simulink model "model_Zbiornik_wsk"  (R2015a)
settings: Solver=ode4  StartTime=0.0  StopTime=100.0  FixedStep=0.01  RelTol=1e-3
values from neighbouring files (symbols this model uses):
  h0 = 20    [NastawyLQR.m]    (also in SzukanieNastaw.m; wskaznikJakosci.m)
  pompaP1 = p1    [SzukanieNastaw.m]
  pompaPWM = ur(1)    [NastawyLQR.m]    (also in SzukanieNastaw.m; SzukanieStanuUstalonego.m = Nastawy(1); wskaznikJakosci.m = params(1))
  ref = 20    [wskaznikJakosci.m]
  zaworP1 = [-49.1428571429 99.1142857143 -23.37]    [parametryWielomianuPWMZaworu.mat]
  zaworPWM = ur(2)    [NastawyLQR.m]    (also in SzukanieNastaw.m; SzukanieStanuUstalonego.m = Nastawy(2); wskaznikJakosci.m = params(2))
undefined symbols (not defined in the file or in its folder): zaworC1, zaworC2
settings Model: Creator=konra  LastModifiedBy=konra

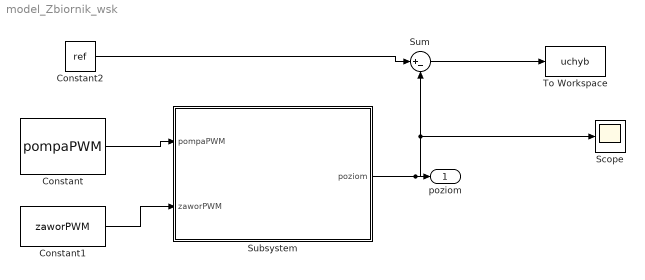
== system model_Zbiornik_wsk ==
  Constant : Constant  Value=pompaPWM
  Constant1 : Constant  Value=zaworPWM
  Constant2 : Constant  Value=ref
  Scope : Scope
      settings: TimeRange=49.99  YMin=19.999999925  YMax=19.999999965
  Subsystem : Subsystem
  Sum : Sum  Inputs=|+-
  To Workspace : ToWorkspace  VariableName=uchyb  SaveFormat=Structure With Time  SampleTime=-1
  poziom : Outport
  wires:
  Subsystem/1(poziom) -> Sum/2, Scope/1, poziom/1
  Constant/1 -> Subsystem/1(pompaPWM)
  Constant1/1 -> Subsystem/2(zaworPWM)
  Constant2/1 -> Sum/1
  Sum/1 -> To Workspace/1

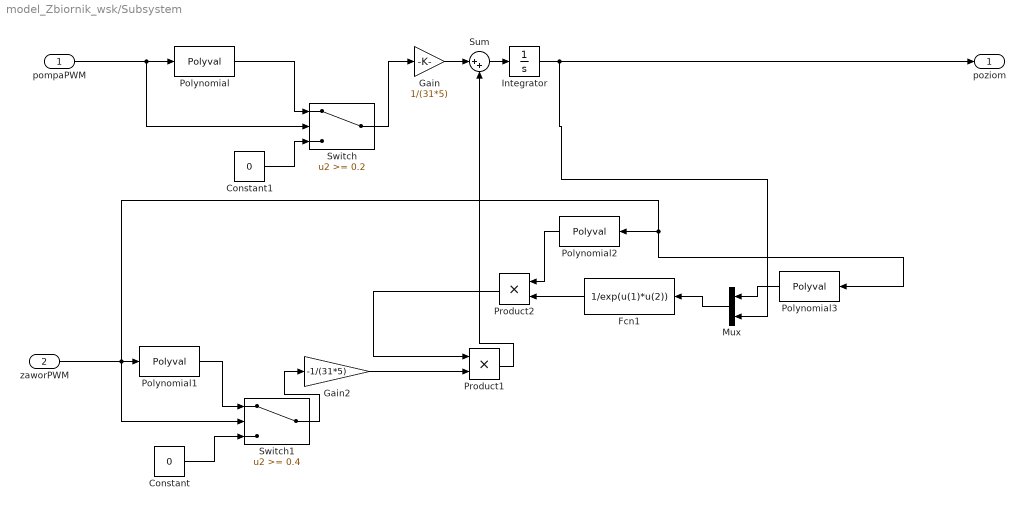
== system model_Zbiornik_wsk/Subsystem ==
  pompaPWM : Inport
  zaworPWM : Inport  Port=2
  Constant : Constant  Value=0
  Constant1 : Constant  Value=0
  Fcn1 : Fcn  Expr=1/exp(u(1)*u(2))
  Gain : Gain  Gain=1/(31*5)
  Gain2 : Gain  Gain=-1/(31*5)
  Integrator : Integrator  InitialCondition=h0
  Mux : Mux  Inputs=2
  Polynomial : Polyval  Coefs=pompaP1
  Polynomial1 : Polyval  Coefs=zaworP1
  Polynomial2 : Polyval  Coefs=zaworC2
  Polynomial3 : Polyval  Coefs=zaworC1
  Product1 : Product
  Product2 : Product
  Sum : Sum  Inputs=|++
  Switch : Switch  Threshold=0.2
  Switch1 : Switch  Threshold=0.4
  poziom : Outport
  wires:
  Switch1/1 -> Gain2/1
  Polynomial1/1 -> Switch1/1
  Constant/1 -> Switch1/3
  Polynomial/1 -> Switch/1
  Constant1/1 -> Switch/3
  Switch/1 -> Gain/1
  pompaPWM/1 -> Switch/2, Polynomial/1
  Gain2/1 -> Product1/2
  Product1/1 -> Sum/2
  Product2/1 -> Product1/1
  Integrator/1 -> poziom/1, Mux/2
  Fcn1/1 -> Product2/2
  zaworPWM/1 -> Switch1/2, Polynomial1/1, Polynomial3/1, Polynomial2/1
  Polynomial2/1 -> Product2/1
  Mux/1 -> Fcn1/1
  Polynomial3/1 -> Mux/1
  Gain/1 -> Sum/1
  Sum/1 -> Integrator/1
